simulink model "DiagramaBloques"  (R2014a)
settings: Solver=ode45  StartTime=0.0  StopTime=100  RelTol=1e-3
PreLoadFcn:
  | variables
InitFcn:
  | eval('variables');
  | variables
StartFcn:
  | variables
settings Model: Creator=jhoan  LastModifiedBy=jhoan

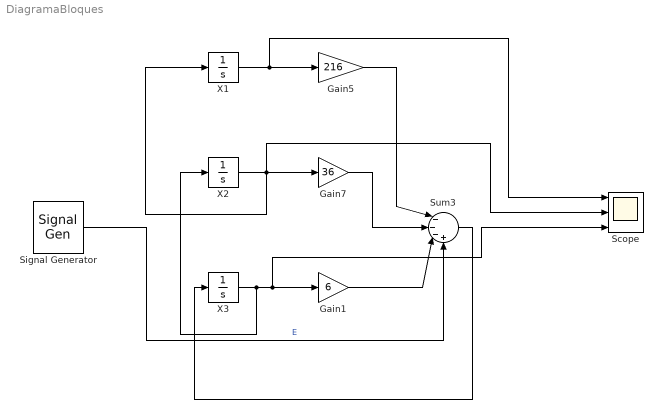
== system DiagramaBloques ==
  Gain1 : Gain  Gain=6
  Gain5 : Gain  Gain=216
  Gain7 : Gain  Gain=36
  Scope : Scope  NumInputPorts=3
      settings: YMin=-5~-5~-5  YMax=5~5~5  SaveName=subSimulink
  Signal Generator : SignalGenerator  WaveForm=square  Amplitude=2  Frequency=10
  Sum3 : Sum  Inputs=|---+
  X1 : Integrator
  X2 : Integrator
  "X3 " : Integrator
  wires:
  "X3 "/1 -> X2/1, Scope/3, Gain1/1
  Gain5/1 -> Sum3/1
  Gain7/1 -> Sum3/2
  Gain1/1 -> Sum3/3
  Signal Generator/1 -> Sum3/4  "E"
  Sum3/1 -> "X3 "/1
  X2/1 -> X1/1, Scope/2, Gain7/1
  X1/1 -> Scope/1, Gain5/1
